simulink model "DEF_2GFL_Eugenie"  (R2022b)
settings: Solver=FixedStepAuto  StartTime=0  StopTime=10  FixedStep=Ts  RelTol=1e-3
undefined symbols (not defined in the file or in its folder): ApparatusDiscreDamping, ApparatusPara, ApparatusPowerFlow, ApparatusType, OtherInputs, PowerFlow, Sbase, Ts, Vbase, Wbase, x_e, Ybase, Zbase
libraries: SimplusGT x10, spsGroundLib x5, spsThreePhaseSeriesRLCBranchLib x4, spsSawtoothGeneratorLib x4, spsabctoAlphaBetaZeroLib x4, spsControlledCurrentSourceLib x3, spsCurrentMeasurementLib x3, spsVoltageMeasurementLib x3, spsThreePhaseParallelRLCBranchLib x2, sps_lib x1
(part 1 of 2)
settings Model: Creator=Maurice  LastModifiedBy=yz34218

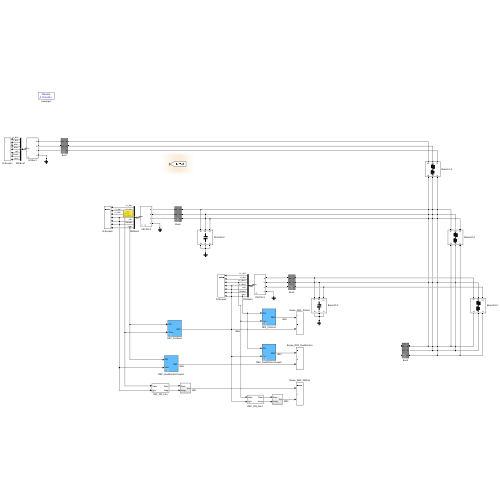
[thumbnail: Simulink's stored preview of the top-level diagram]
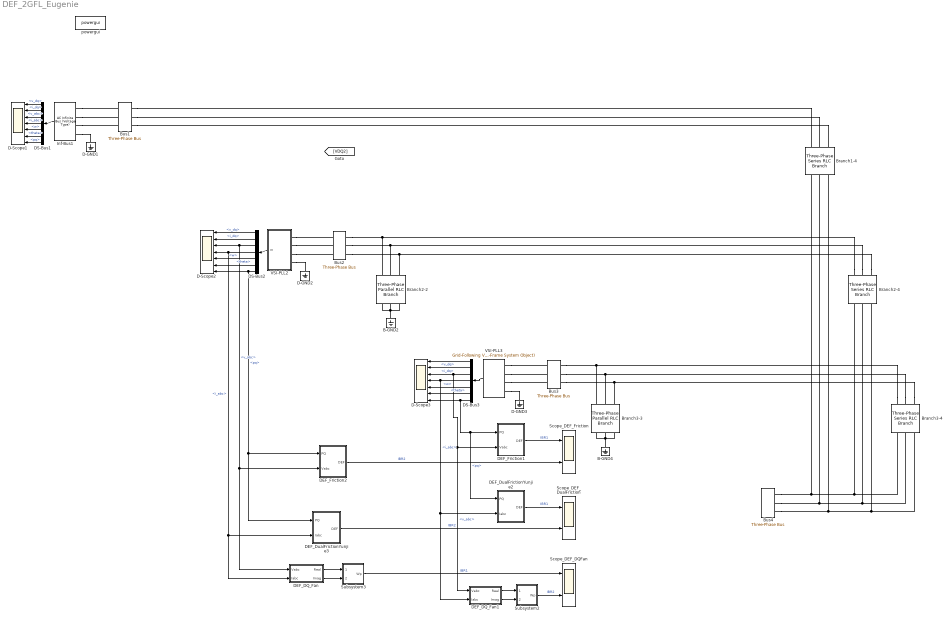
== system DEF_2GFL_Eugenie ==
  B-GND2 : spsGroundLib/Ground  LConnTagsString=a
  B-GND4 : spsGroundLib/Ground  LConnTagsString=a
  Branch1-4 : spsThreePhaseSeriesRLCBranchLib/Three-Phase Series RLC Branch  LConnTagsString=A|B|C  RConnTagsString=A|B|C  BranchType=RL  Resistance=(0.017)*Zbase  Inductance=(0.170)*Zbase/Wbase  Capacitance=1e-6  Measurements=None
  Branch2-2 : spsThreePhaseParallelRLCBranchLib/Three-Phase Parallel RLC Branch  LConnTagsString=A|B|C  RConnTagsString=A|B|C  BranchType=C  Resistance=(Inf)*Zbase  Inductance=(Inf)*Zbase/Wbase  Capacitance=(0.3)*Ybase/Wbase  Measurements=None
  Branch2-4 : spsThreePhaseSeriesRLCBranchLib/Three-Phase Series RLC Branch  LConnTagsString=A|B|C  RConnTagsString=A|B|C  BranchType=RL  Resistance=(0.005)*Zbase  Inductance=(0.05)*Zbase/Wbase  Capacitance=1e-6  Measurements=None
  Branch3-3 : spsThreePhaseParallelRLCBranchLib/Three-Phase Parallel RLC Branch  LConnTagsString=A|B|C  RConnTagsString=A|B|C  BranchType=C  Resistance=(Inf)*Zbase  Inductance=(Inf)*Zbase/Wbase  Capacitance=(0.3)*Ybase/Wbase  Measurements=None
  Branch3-4 : spsThreePhaseSeriesRLCBranchLib/Three-Phase Series RLC Branch  LConnTagsString=A|B|C  RConnTagsString=A|B|C  BranchType=RL  Resistance=(0.005)*Zbase  Inductance=(0.05)*Zbase/Wbase  Capacitance=1e-6  Measurements=None
  Bus{1..4} (4 alike) : SimplusGT/Three-Phase Bus  Vbase=1  Sbase=1
      settings: SourceProductName=Simplus Grid Tool
  D-GND1 : spsGroundLib/Ground  LConnTagsString=a
  D-GND2 : spsGroundLib/Ground  LConnTagsString=a
  D-GND3 : spsGroundLib/Ground  LConnTagsString=a
  D-Scope1 : Scope  NumInputPorts=7
  D-Scope2 : Scope  NumInputPorts=7
  D-Scope3 : Scope  NumInputPorts=7
  DEF_DQ_Fan : Subsystem  mask{PowerFlow_App=ApparatusPowerFlow{2}}
      mask prompts: PowerFlow_App "Power Flow"
  DEF_DQ_Fan1 : Subsystem  mask{PowerFlow_App=ApparatusPowerFlow{3}}
      mask prompts: PowerFlow_App "Power Flow"
  DEF_DualFrictionYunjie2 : Subsystem  mask{PowerFlow_App=ApparatusPowerFlow{3}}
      mask prompts: PowerFlow_App "Power Flow"
  DEF_DualFrictionYunjie3 : Subsystem  mask{PowerFlow_App=ApparatusPowerFlow{3}}
      mask prompts: PowerFlow_App "Power Flow"
  DEF_Friction1 : Subsystem  mask{PowerFlow_App=ApparatusPowerFlow{3}}
      mask prompts: PowerFlow_App "Power Flow"
  DEF_Friction2 : Subsystem  mask{PowerFlow_App=ApparatusPowerFlow{2}}
      mask prompts: PowerFlow_App "Power Flow"
  DS-Bus1 : BusSelector  OutputSignals=v_dq,i_dq,v_abc,i_abc,w,theta,pq
  DS-Bus2 : BusSelector  OutputSignals=v_dq,i_dq,v_abc,i_abc,w,theta,pq
  DS-Bus3 : BusSelector  OutputSignals=v_dq,i_dq,v_abc,i_abc,w,theta,pq
  Inf-Bus1 : SimplusGT/AC Infinite Bus (Voltage Type)  Ts=Ts  Sbase=Sbase  Vbase=Vbase  Wbase=Wbase  vd=PowerFlow{1}(3)  vq=0  theta0=PowerFlow{1}(4)  w=Wbase  R=1e-30
      settings: SourceProductName=Simplus Grid Tool
  Scope_DEF_DQFan : Scope  NumInputPorts=2
  Scope_DEF_DualFriction : Scope  NumInputPorts=2
  Scope_DEF_Friction : Scope  NumInputPorts=2
  Subsystem2 : Subsystem
  Subsystem3 : Subsystem
  VSI-PLL2 : Subsystem  AncestorBlock=|  mask{Ts=Ts, Sbase=Sbase, Vbase=Vbase, Wbase=Wbase, ApparatusType=ApparatusType{2}, ApparatusPara=ApparatusPara{2}, PowerFlow=ApparatusPowerFlow{2}, x0=x_e{2}, OtherInputs=OtherInputs{2}, DiscreMethod=Hybrid Trapezoidal, EnableInsideModification=off, DiscreDampingFlag=on, DiscreDampingValue=ApparatusDiscreDamping{2}, LinearizationTimes=1, DirectFeedthrough=off}
      | SimplusGT/Grid-Following
      | Voltage-Source Inverter
      | (dq-Frame System Object)
      mask prompts: Ts "Ts (s), samping period"; Sbase "Sbase (VA), power base"; Vbase "Vbase (V), voltage base"; Wbase "Wbase (rad/s), frequency base"; ApparatusType "Apparatus type"; ApparatusPara "Apparatus parameters"; PowerFlow "Power flow parameters"; x0 "x0, initial states"; OtherInputs "Other inputs"; DiscreMethod "Discretization method"; EnableInsideModification "Enable inside modification"; DiscreDampingFlag "Enable discretization damping"; DiscreDampingValue "Discretization damping value"; LinearizationTimes "Linearization times"; DirectFeedthrough "Direct feedthrough"
      mask init:
      | SimplusGT.Simulink.DeviceMaskInitialization(EnableInsideModification,DiscreDampingFlag);
      settings: LibrarySourceBlock=|
      | SimplusGT/Grid-Following
      | Voltage-Source Inverter
      | (dq-Frame System Object)
      mask TypeOptions DiscreMethod: Forward Euler | Hybrid Trapezoidal | Virtual Damping
      mask TypeOptions LinearizationTimes: 1 | 2
  VSI-PLL3 : SimplusGT/Grid-Following Voltage-Source Inverter (dq-Frame System Object)  Ts=Ts  Sbase=Sbase  Vbase=Vbase  Wbase=Wbase  ApparatusType=ApparatusType{3}  ApparatusPara=ApparatusPara{3}  PowerFlow=ApparatusPowerFlow{3}  x0=x_e{3}  OtherInputs=OtherInputs{3}  DiscreMethod=Hybrid Trapezoidal  EnableInsideModification=off  DiscreDampingFlag=on  DiscreDampingValue=ApparatusDiscreDamping{3}  LinearizationTimes=1  DirectFeedthrough=off
      settings: SourceProductName=Simplus Grid Tool
  powergui : sps_lib/powergui  Priority=1  SimulationMode=Discrete  SampleTime=Ts  frequency=60  Iterations=50  frequencyindice=0  Pbase=100e6  ErrMax=1e-4  UnitsV=kV  UnitsW=MW  buscounter=0  FunctionMessages=off  echomessages=off  EnableUseOfTLC=off  CurrentSourceSwitches=off  DisableSnubberDevices=off  DisableRonSwitches=off  DisableVfSwitches=off  DisplayEquations=off  AutomaticDiscreteSolvers=off  SolverType=Tustin/Backward Euler (TBE)  Interpol=off  ExternalGateDelay=off  methode=off  Ts=100  x0status=blocks  SPID=on  SwTol=0  HookPort=off  NonlinearTolerance=1e-4  nMaxIteration=100  ContinueOnMaxIteration=off  RestoreLinks=warning  ResistiveCurrentMeasurement=off  Frange=[0:2:500]  Ylog=off  Xlog=on  ShowGrid=off  save=off  variable=ZData  structure=0  ZoomFFT=off  StartTime=0.0  cycles=1  DisplayStyle=1  fundamental=60  FreqAxis=off  MaxFrequency=1000  frequencyindicesteady=1  RmsSteady=1  display=off
  wires:
  Inf-Bus1/1 -> DS-Bus1/1
  DS-Bus1/1 -> D-Scope1/1  "<v_dq>"
  DS-Bus1/2 -> D-Scope1/2  "<i_dq>"
  DS-Bus1/3 -> D-Scope1/3  "<v_abc>"
  DS-Bus1/4 -> D-Scope1/4  "<i_abc>"
  DS-Bus1/5 -> D-Scope1/5  "<w>"
  DS-Bus1/6 -> D-Scope1/6  "<theta>"
  DS-Bus1/7 -> D-Scope1/7  "<pq>"
  DS-Bus2/3 -> DEF_Friction2/2(Vabc), DEF_DQ_Fan/1(Vabc), D-Scope2/3  "<v_abc>"
  DS-Bus2/4 -> DEF_DualFrictionYunjie3/2(Iabc), DEF_DQ_Fan/2(Iabc), D-Scope2/4  "<i_abc>"
  DS-Bus2/5 -> D-Scope2/5  "<w>"
  DS-Bus2/6 -> D-Scope2/6  "<theta>"
  DS-Bus2/7 -> D-Scope2/7, DEF_Friction2/1(PQ), DEF_DualFrictionYunjie3/1(PQ)  "<pq>"
  VSI-PLL3/1 -> DS-Bus3/1
  DS-Bus3/1 -> D-Scope3/1  "<v_dq>"
  DS-Bus3/2 -> D-Scope3/2  "<i_dq>"
  DS-Bus3/3 -> DEF_Friction1/2(Vabc), DEF_DQ_Fan1/1(Vabc), D-Scope3/3  "<v_abc>"
  DS-Bus3/4 -> DEF_DQ_Fan1/2(Iabc), DEF_DualFrictionYunjie2/2(Iabc), D-Scope3/4  "<i_abc>"
  DS-Bus3/5 -> D-Scope3/5  "<w>"
  DS-Bus3/6 -> D-Scope3/6  "<theta>"
  DS-Bus3/7 -> DEF_DualFrictionYunjie2/1(PQ), DEF_Friction1/1(PQ), D-Scope3/7  "<pq>"
  DEF_Friction1/1(DEF) -> Scope_DEF_Friction/1  "IBR1"
  DEF_Friction2/1(DEF) -> Scope_DEF_Friction/2  "IBR2"
  DEF_DualFrictionYunjie2/1(DEF) -> Scope_DEF_DualFriction/1  "IBR1"
  DEF_DualFrictionYunjie3/1(DEF) -> Scope_DEF_DualFriction/2  "IBR2"
  DS-Bus2/2 -> D-Scope2/2  "<i_dq>"
  DS-Bus2/1 -> D-Scope2/1  "<v_dq>"
  DEF_DQ_Fan1/1(Real) -> Subsystem2/1(Real)
  DEF_DQ_Fan1/2(Imag) -> Subsystem2/2(Imag)
  Subsystem2/1(Wp) -> Scope_DEF_DQFan/2  "IBR2"
  DEF_DQ_Fan/2(Imag) -> Subsystem3/2(Imag)
  DEF_DQ_Fan/1(Real) -> Subsystem3/1(Real)
  Subsystem3/1(Wp) -> Scope_DEF_DQFan/1  "IBR1"
  VSI-PLL2/1(m) -> DS-Bus2/1
  connections:
  Inf-Bus1/LConn4 -- D-GND1/LConn1
  VSI-PLL2/LConn4 -- D-GND2/LConn1
  VSI-PLL3/LConn4 -- D-GND3/LConn1
  Branch2-2/RConn1 -- Branch2-2/RConn2 -- Branch2-2/RConn3 -- B-GND2/LConn1
  Branch3-3/RConn1 -- Branch3-3/RConn2 -- Branch3-3/RConn3 -- B-GND4/LConn1
  Branch1-4/RConn1 -- Bus4/RConn1 -- Branch3-4/RConn1 -- Branch2-4/RConn1
  Branch1-4/RConn2 -- Bus4/RConn2 -- Branch3-4/RConn2 -- Branch2-4/RConn2
  Branch1-4/RConn3 -- Bus4/RConn3 -- Branch3-4/RConn3 -- Branch2-4/RConn3
  Bus1/RConn1 -- Branch1-4/LConn1
  Bus1/RConn2 -- Branch1-4/LConn2
  Bus1/RConn3 -- Branch1-4/LConn3
  Branch2-4/LConn1 -- Bus2/RConn1 -- Branch2-2/LConn1
  Branch2-4/LConn2 -- Bus2/RConn2 -- Branch2-2/LConn2
  Branch2-4/LConn3 -- Bus2/RConn3 -- Branch2-2/LConn3
  Branch3-4/LConn1 -- Bus3/RConn1 -- Branch3-3/LConn1
  Branch3-4/LConn2 -- Bus3/RConn2 -- Branch3-3/LConn2
  Branch3-4/LConn3 -- Bus3/RConn3 -- Branch3-3/LConn3
  Inf-Bus1/LConn1 -- Bus1/LConn1
  Inf-Bus1/LConn2 -- Bus1/LConn2
  Inf-Bus1/LConn3 -- Bus1/LConn3
  VSI-PLL2/LConn1 -- Bus2/LConn1
  VSI-PLL2/LConn2 -- Bus2/LConn2
  VSI-PLL2/LConn3 -- Bus2/LConn3
  VSI-PLL3/LConn1 -- Bus3/LConn1
  VSI-PLL3/LConn2 -- Bus3/LConn2
  VSI-PLL3/LConn3 -- Bus3/LConn3

== system DEF_2GFL_Eugenie/DEF_DQ_Fan ==
  Vabc : Inport
  Iabc : Inport  Port=2
  DEF_DualFrictionFan2 : Subsystem
  Mux : Mux  Inputs=2
  Mux1 : Mux  Inputs=2
  dq2DQ : Subsystem
  dq2DQ1 : Subsystem
  Real : Outport
  Imag : Outport  Port=2
  wires:
  Vabc/1 -> dq2DQ/1(abc)
  Iabc/1 -> dq2DQ1/1(abc)
  dq2DQ/1(D) -> Mux/1
  dq2DQ/2(Q) -> Mux/2
  dq2DQ1/1(D) -> Mux1/1
  dq2DQ1/2(Q) -> Mux1/2
  Mux1/1 -> DEF_DualFrictionFan2/2(IDQ)
  Mux/1 -> DEF_DualFrictionFan2/1(VDQ)
  DEF_DualFrictionFan2/1(Real) -> Real/1
  DEF_DualFrictionFan2/2(Imag) -> Imag/1

== system DEF_2GFL_Eugenie/DEF_DQ_Fan1 ==
  Vabc : Inport
  Iabc : Inport  Port=2
  DEF_DualFrictionFan2 : Subsystem
  Mux : Mux  Inputs=2
  Mux1 : Mux  Inputs=2
  dq2DQ : Subsystem
  dq2DQ1 : Subsystem
  Real : Outport
  Imag : Outport  Port=2
  wires:
  DEF_DualFrictionFan2/2(Imag) -> Imag/1
  DEF_DualFrictionFan2/1(Real) -> Real/1
  Mux/1 -> DEF_DualFrictionFan2/1(VDQ)
  Mux1/1 -> DEF_DualFrictionFan2/2(IDQ)
  dq2DQ1/2(Q) -> Mux1/2
  dq2DQ1/1(D) -> Mux1/1
  dq2DQ/2(Q) -> Mux/2
  dq2DQ/1(D) -> Mux/1
  Iabc/1 -> dq2DQ1/1(abc)
  Vabc/1 -> dq2DQ/1(abc)

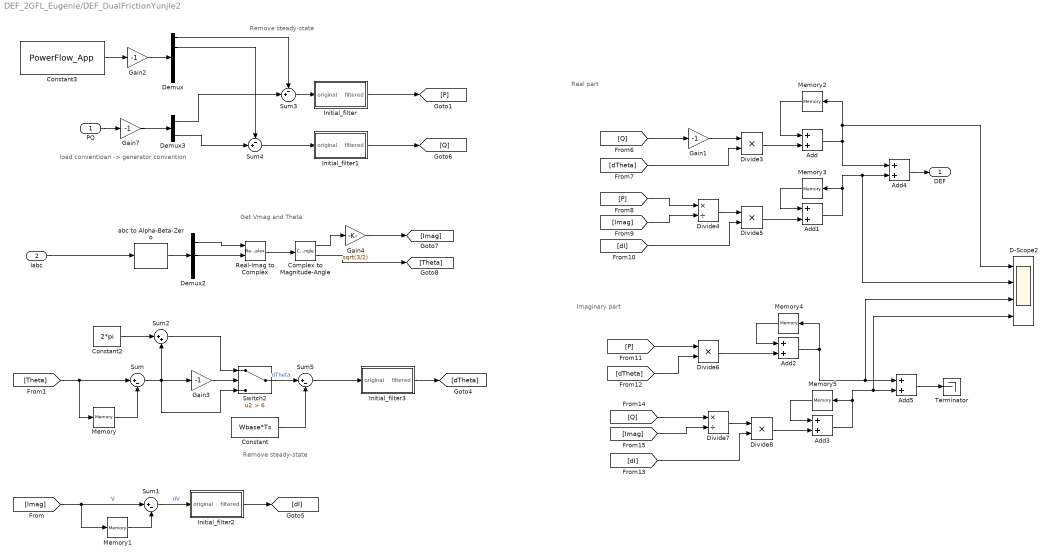
== system DEF_2GFL_Eugenie/DEF_DualFrictionYunjie2 ==
  note: Real part
  note: Imaginary part
  note: load conventioan -> generator convention
  note: Remove steady-state
  note: Remove steady-state
  note: Get Vmag and Theta
  PQ : Inport
  Iabc : Inport  Port=2
  Add{,1..5} (6 alike) : Sum
  Complex to Magnitude-Angle : ComplexToMagnitudeAngle
  Constant : Constant  Value=Wbase*Ts
  Constant2 : Constant  Value=2*pi
  Constant3 : Constant  Value=PowerFlow_App
  D-Scope2 : Scope  NumInputPorts=4
  Demux : Demux  Outputs=5
  Demux2 : Demux  Outputs=3
  Demux3 : Demux  Outputs=2
  Divide{3,5..6,8} (4 alike) : Product  Inputs=**
  Divide4 : Product  Inputs=*/
  Divide7 : Product  Inputs=*/
  Gain{1..3,7} (4 alike) : Gain  Gain=-1
  Gain4 : Gain  Gain=sqrt(3/2)
  Initial_filter : Subsystem
  Initial_filter1 : Subsystem
  Initial_filter2 : Subsystem
  Initial_filter3 : Subsystem
  Memory{,1..5} (6 alike) : Memory
  Real-Imag to Complex : RealImagToComplex
  Sum : Sum  Inputs=|+-
  Sum1 : Sum  Inputs=|+-
  Sum2 : Sum  Inputs=|++
  Sum3 : Sum  Inputs=-+|
  Sum4 : Sum  Inputs=-+|
  Sum5 : Sum  Inputs=|+-
  Switch2 : Switch  Criteria=u2 > Threshold  Threshold=6  SaturateOnIntegerOverflow=off  InputSameDT=off
  Terminator : Terminator
  abc to Alpha-Beta-Zero : spsabctoAlphaBetaZeroLib/abc to Alpha-Beta-Zero
  DEF : Outport
  wires:
  Add4/1 -> DEF/1
  Add5/1 -> Terminator/1
  [Q] -> Divide7/1
  [Imag] -> Divide4/2
  Divide3/1 -> Add/2
  [P] -> Divide4/1
  [Q] -> Gain1/1
  Gain1/1 -> Divide3/1
  [dTheta] -> Divide3/2
  [dI] -> Divide5/2
  [P] -> Divide6/1
  Divide4/1 -> Divide5/1
  [dTheta] -> Divide6/2
  [dI] -> Divide8/2
  Divide7/1 -> Divide8/1
  [Imag] -> Divide7/2
  Memory1/1 -> Sum1/2
  [Imag] -> Memory1/1, Sum1/1  "V"
  Sum1/1 -> Initial_filter2/1(original)  "dV"
  [Theta] -> Sum/1, Memory/1
  Add/1 -> D-Scope2/1, Memory2/1, Add4/1
  Memory2/1 -> Add/1
  Divide5/1 -> Add1/2
  Memory3/1 -> Add1/1
  Memory4/1 -> Add2/1
  Add2/1 -> D-Scope2/3, Add5/1, Memory4/1
  Divide6/1 -> Add2/2
  Memory5/1 -> Add3/1
  Add3/1 -> D-Scope2/4, Add5/2, Memory5/1
  Divide8/1 -> Add3/2
  Iabc/1 -> abc to Alpha-Beta-Zero/1
  abc to Alpha-Beta-Zero/1 -> Demux2/1
  Memory/1 -> Sum/2
  Sum/1 -> Gain3/1, Switch2/3, Sum2/2
  Sum2/1 -> Switch2/1
  Constant2/1 -> Sum2/1
  Gain3/1 -> Switch2/2
  Constant3/1 -> Gain2/1
  Sum3/1 -> Initial_filter/1(original)
  Demux/1 -> Sum3/1
  Sum4/1 -> Initial_filter1/1(original)
  Demux/2 -> Sum4/1
  Demux3/1 -> Sum3/2
  Demux3/2 -> Sum4/2
  PQ/1 -> Gain7/1
  Initial_filter/1(filtered) -> [P]
  Initial_filter1/1(filtered) -> [Q]
  Initial_filter2/1(filtered) -> [dI]
  Initial_filter3/1(filtered) -> [dTheta]
  Complex to Magnitude-Angle/2 -> [Theta]
  Gain4/1 -> [Imag]
  Complex to Magnitude-Angle/1 -> Gain4/1
  Real-Imag to Complex/1 -> Complex to Magnitude-Angle/1
  Demux2/1 -> Real-Imag to Complex/1
  Demux2/2 -> Real-Imag to Complex/2
  Gain2/1 -> Demux/1
  Gain7/1 -> Demux3/1
  Switch2/1 -> Sum5/1  "dTheta"
  Sum5/1 -> Initial_filter3/1(original)
  Constant/1 -> Sum5/2
  Add1/1 -> D-Scope2/2, Add4/2, Memory3/1

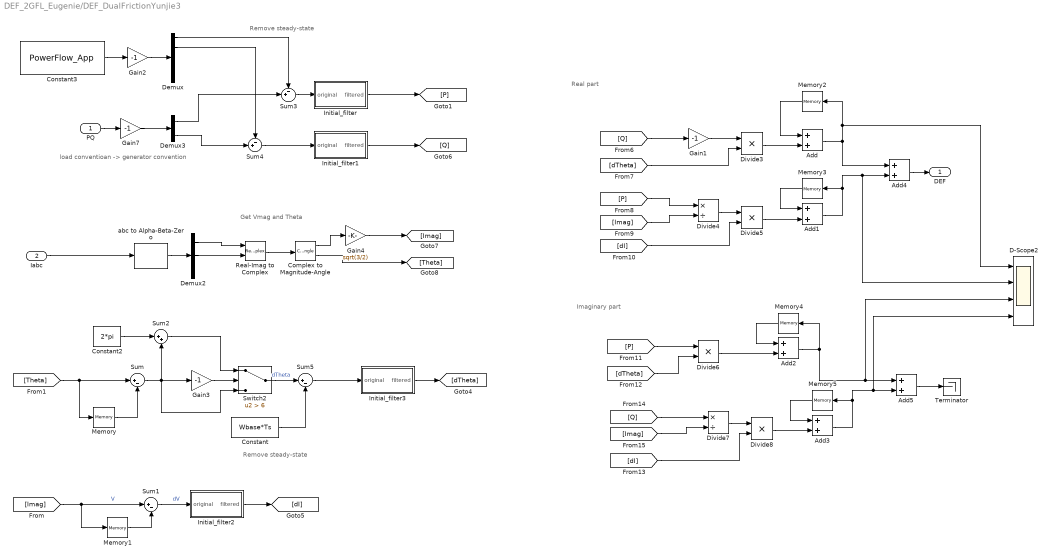
== system DEF_2GFL_Eugenie/DEF_DualFrictionYunjie3 ==
  note: Real part
  note: Imaginary part
  note: load conventioan -> generator convention
  note: Remove steady-state
  note: Remove steady-state
  note: Get Vmag and Theta
  PQ : Inport
  Iabc : Inport  Port=2
  Add{,1..5} (6 alike) : Sum
  Complex to Magnitude-Angle : ComplexToMagnitudeAngle
  Constant : Constant  Value=Wbase*Ts
  Constant2 : Constant  Value=2*pi
  Constant3 : Constant  Value=PowerFlow_App
  D-Scope2 : Scope  NumInputPorts=4
  Demux : Demux  Outputs=5
  Demux2 : Demux  Outputs=3
  Demux3 : Demux  Outputs=2
  Divide{3,5..6,8} (4 alike) : Product  Inputs=**
  Divide4 : Product  Inputs=*/
  Divide7 : Product  Inputs=*/
  Gain{1..3,7} (4 alike) : Gain  Gain=-1
  Gain4 : Gain  Gain=sqrt(3/2)
  Initial_filter : Subsystem
  Initial_filter1 : Subsystem
  Initial_filter2 : Subsystem
  Initial_filter3 : Subsystem
  Memory{,1..5} (6 alike) : Memory
  Real-Imag to Complex : RealImagToComplex
  Sum : Sum  Inputs=|+-
  Sum1 : Sum  Inputs=|+-
  Sum2 : Sum  Inputs=|++
  Sum3 : Sum  Inputs=-+|
  Sum4 : Sum  Inputs=-+|
  Sum5 : Sum  Inputs=|+-
  Switch2 : Switch  Criteria=u2 > Threshold  Threshold=6  SaturateOnIntegerOverflow=off  InputSameDT=off
  Terminator : Terminator
  abc to Alpha-Beta-Zero : spsabctoAlphaBetaZeroLib/abc to Alpha-Beta-Zero
  DEF : Outport
  wires:
  Add4/1 -> DEF/1
  Add5/1 -> Terminator/1
  [Q] -> Divide7/1
  [Imag] -> Divide4/2
  Divide3/1 -> Add/2
  [P] -> Divide4/1
  [Q] -> Gain1/1
  Gain1/1 -> Divide3/1
  [dTheta] -> Divide3/2
  [dI] -> Divide5/2
  [P] -> Divide6/1
  Divide4/1 -> Divide5/1
  [dTheta] -> Divide6/2
  [dI] -> Divide8/2
  Divide7/1 -> Divide8/1
  [Imag] -> Divide7/2
  Memory1/1 -> Sum1/2
  [Imag] -> Memory1/1, Sum1/1  "V"
  Sum1/1 -> Initial_filter2/1(original)  "dV"
  [Theta] -> Sum/1, Memory/1
  Add/1 -> D-Scope2/1, Memory2/1, Add4/1
  Memory2/1 -> Add/1
  Divide5/1 -> Add1/2
  Memory3/1 -> Add1/1
  Memory4/1 -> Add2/1
  Add2/1 -> D-Scope2/3, Add5/1, Memory4/1
  Divide6/1 -> Add2/2
  Memory5/1 -> Add3/1
  Add3/1 -> D-Scope2/4, Add5/2, Memory5/1
  Divide8/1 -> Add3/2
  Iabc/1 -> abc to Alpha-Beta-Zero/1
  abc to Alpha-Beta-Zero/1 -> Demux2/1
  Memory/1 -> Sum/2
  Sum/1 -> Gain3/1, Switch2/3, Sum2/2
  Sum2/1 -> Switch2/1
  Constant2/1 -> Sum2/1
  Gain3/1 -> Switch2/2
  Constant3/1 -> Gain2/1
  Sum3/1 -> Initial_filter/1(original)
  Demux/1 -> Sum3/1
  Sum4/1 -> Initial_filter1/1(original)
  Demux/2 -> Sum4/1
  Demux3/1 -> Sum3/2
  Demux3/2 -> Sum4/2
  PQ/1 -> Gain7/1
  Initial_filter/1(filtered) -> [P]
  Initial_filter1/1(filtered) -> [Q]
  Initial_filter2/1(filtered) -> [dI]
  Initial_filter3/1(filtered) -> [dTheta]
  Complex to Magnitude-Angle/2 -> [Theta]
  Gain4/1 -> [Imag]
  Complex to Magnitude-Angle/1 -> Gain4/1
  Real-Imag to Complex/1 -> Complex to Magnitude-Angle/1
  Demux2/1 -> Real-Imag to Complex/1
  Demux2/2 -> Real-Imag to Complex/2
  Gain2/1 -> Demux/1
  Gain7/1 -> Demux3/1
  Switch2/1 -> Sum5/1  "dTheta"
  Sum5/1 -> Initial_filter3/1(original)
  Constant/1 -> Sum5/2
  Add1/1 -> D-Scope2/2, Add4/2, Memory3/1

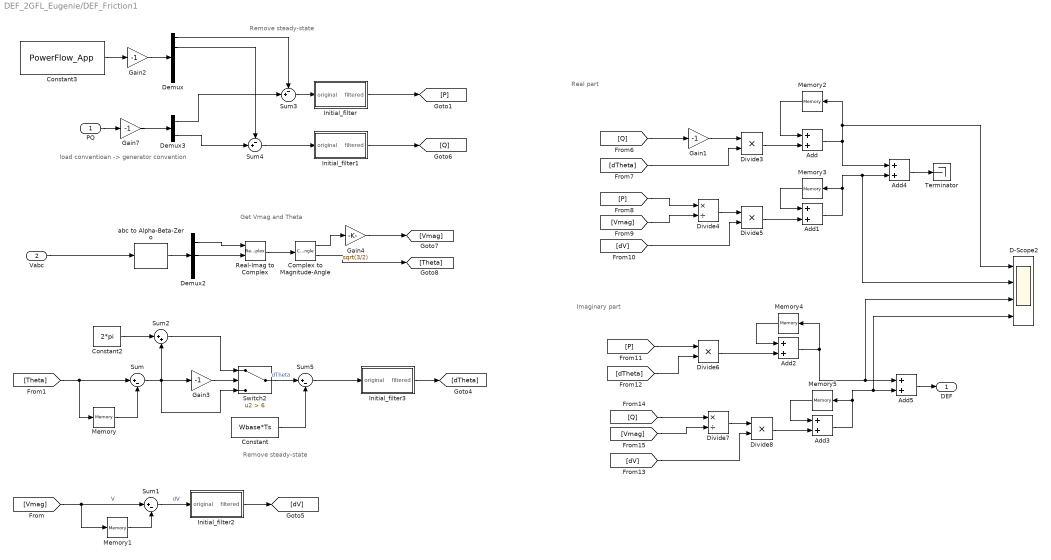
== system DEF_2GFL_Eugenie/DEF_Friction1 ==
  note: Get Vmag and Theta
  note: Remove steady-state
  note: Remove steady-state
  note: load conventioan -> generator convention
  note: Imaginary part
  note: Real part
  PQ : Inport
  Vabc : Inport  Port=2
  Add{,1..5} (6 alike) : Sum
  Complex to Magnitude-Angle : ComplexToMagnitudeAngle
  Constant : Constant  Value=Wbase*Ts
  Constant2 : Constant  Value=2*pi
  Constant3 : Constant  Value=PowerFlow_App
  D-Scope2 : Scope  NumInputPorts=4
  Demux : Demux  Outputs=5
  Demux2 : Demux  Outputs=3
  Demux3 : Demux  Outputs=2
  Divide{3,5..6,8} (4 alike) : Product  Inputs=**
  Divide4 : Product  Inputs=*/
  Divide7 : Product  Inputs=*/
  Gain{1..3,7} (4 alike) : Gain  Gain=-1
  Gain4 : Gain  Gain=sqrt(3/2)
  Initial_filter : Subsystem
  Initial_filter1 : Subsystem
  Initial_filter2 : Subsystem
  Initial_filter3 : Subsystem
  Memory{,1..5} (6 alike) : Memory
  Real-Imag to Complex : RealImagToComplex
  Sum : Sum  Inputs=|+-
  Sum1 : Sum  Inputs=|+-
  Sum2 : Sum  Inputs=|++
  Sum3 : Sum  Inputs=-+|
  Sum4 : Sum  Inputs=-+|
  Sum5 : Sum  Inputs=|+-
  Switch2 : Switch  Criteria=u2 > Threshold  Threshold=6  SaturateOnIntegerOverflow=off  InputSameDT=off
  Terminator : Terminator
  abc to Alpha-Beta-Zero : spsabctoAlphaBetaZeroLib/abc to Alpha-Beta-Zero
  DEF : Outport
  wires:
  Add1/1 -> Memory3/1, Add4/2, D-Scope2/2
  Add4/1 -> Terminator/1
  Add5/1 -> DEF/1
  Constant/1 -> Sum5/2
  Sum5/1 -> Initial_filter3/1(original)
  Switch2/1 -> Sum5/1  "dTheta"
  Gain7/1 -> Demux3/1
  Gain2/1 -> Demux/1
  Demux2/2 -> Real-Imag to Complex/2
  Demux2/1 -> Real-Imag to Complex/1
  Real-Imag to Complex/1 -> Complex to Magnitude-Angle/1
  Complex to Magnitude-Angle/1 -> Gain4/1
  Gain4/1 -> [Vmag]
  Complex to Magnitude-Angle/2 -> [Theta]
  Initial_filter3/1(filtered) -> [dTheta]
  Initial_filter2/1(filtered) -> [dV]
  Initial_filter1/1(filtered) -> [Q]
  Initial_filter/1(filtered) -> [P]
  PQ/1 -> Gain7/1
  Demux3/2 -> Sum4/2
  Demux3/1 -> Sum3/2
  Demux/2 -> Sum4/1
  Sum4/1 -> Initial_filter1/1(original)
  Demux/1 -> Sum3/1
  Sum3/1 -> Initial_filter/1(original)
  Constant3/1 -> Gain2/1
  Gain3/1 -> Switch2/2
  Constant2/1 -> Sum2/1
  Sum2/1 -> Switch2/1
  Sum/1 -> Sum2/2, Switch2/3, Gain3/1
  Memory/1 -> Sum/2
  abc to Alpha-Beta-Zero/1 -> Demux2/1
  Vabc/1 -> abc to Alpha-Beta-Zero/1
  Divide8/1 -> Add3/2
  Add3/1 -> Memory5/1, Add5/2, D-Scope2/4
  Memory5/1 -> Add3/1
  Divide6/1 -> Add2/2
  Add2/1 -> Memory4/1, Add5/1, D-Scope2/3
  Memory4/1 -> Add2/1
  Memory3/1 -> Add1/1
  Divide5/1 -> Add1/2
  Memory2/1 -> Add/1
  Add/1 -> Add4/1, Memory2/1, D-Scope2/1
  [Theta] -> Memory/1, Sum/1
  Sum1/1 -> Initial_filter2/1(original)  "dV"
  [Vmag] -> Sum1/1, Memory1/1  "V"
  Memory1/1 -> Sum1/2
  [Vmag] -> Divide7/2
  Divide7/1 -> Divide8/1
  [dV] -> Divide8/2
  [dTheta] -> Divide6/2
  Divide4/1 -> Divide5/1
  [P] -> Divide6/1
  [dV] -> Divide5/2
  [dTheta] -> Divide3/2
  Gain1/1 -> Divide3/1
  [Q] -> Gain1/1
  [P] -> Divide4/1
  Divide3/1 -> Add/2
  [Vmag] -> Divide4/2
  [Q] -> Divide7/1

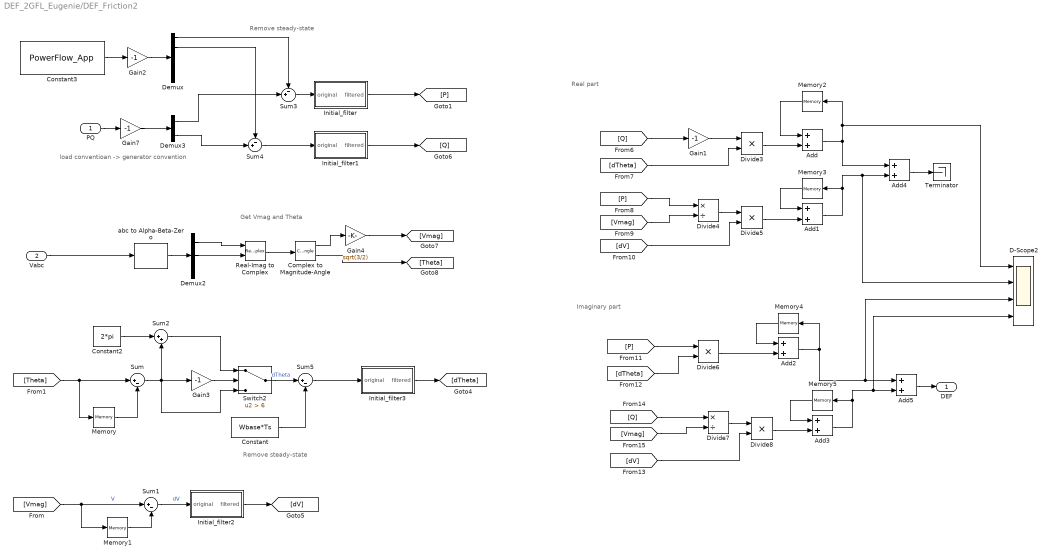
== system DEF_2GFL_Eugenie/DEF_Friction2 ==
  note: Get Vmag and Theta
  note: Remove steady-state
  note: Remove steady-state
  note: load conventioan -> generator convention
  note: Imaginary part
  note: Real part
  PQ : Inport
  Vabc : Inport  Port=2
  Add{,1..5} (6 alike) : Sum
  Complex to Magnitude-Angle : ComplexToMagnitudeAngle
  Constant : Constant  Value=Wbase*Ts
  Constant2 : Constant  Value=2*pi
  Constant3 : Constant  Value=PowerFlow_App
  D-Scope2 : Scope  NumInputPorts=4
  Demux : Demux  Outputs=5
  Demux2 : Demux  Outputs=3
  Demux3 : Demux  Outputs=2
  Divide{3,5..6,8} (4 alike) : Product  Inputs=**
  Divide4 : Product  Inputs=*/
  Divide7 : Product  Inputs=*/
  Gain{1..3,7} (4 alike) : Gain  Gain=-1
  Gain4 : Gain  Gain=sqrt(3/2)
  Initial_filter : Subsystem
  Initial_filter1 : Subsystem
  Initial_filter2 : Subsystem
  Initial_filter3 : Subsystem
  Memory{,1..5} (6 alike) : Memory
  Real-Imag to Complex : RealImagToComplex
  Sum : Sum  Inputs=|+-
  Sum1 : Sum  Inputs=|+-
  Sum2 : Sum  Inputs=|++
  Sum3 : Sum  Inputs=-+|
  Sum4 : Sum  Inputs=-+|
  Sum5 : Sum  Inputs=|+-
  Switch2 : Switch  Criteria=u2 > Threshold  Threshold=6  SaturateOnIntegerOverflow=off  InputSameDT=off
  Terminator : Terminator
  abc to Alpha-Beta-Zero : spsabctoAlphaBetaZeroLib/abc to Alpha-Beta-Zero
  DEF : Outport
  wires:
  Add1/1 -> Memory3/1, Add4/2, D-Scope2/2
  Add4/1 -> Terminator/1
  Add5/1 -> DEF/1
  Constant/1 -> Sum5/2
  Sum5/1 -> Initial_filter3/1(original)
  Switch2/1 -> Sum5/1  "dTheta"
  Gain7/1 -> Demux3/1
  Gain2/1 -> Demux/1
  Demux2/2 -> Real-Imag to Complex/2
  Demux2/1 -> Real-Imag to Complex/1
  Real-Imag to Complex/1 -> Complex to Magnitude-Angle/1
  Complex to Magnitude-Angle/1 -> Gain4/1
  Gain4/1 -> [Vmag]
  Complex to Magnitude-Angle/2 -> [Theta]
  Initial_filter3/1(filtered) -> [dTheta]
  Initial_filter2/1(filtered) -> [dV]
  Initial_filter1/1(filtered) -> [Q]
  Initial_filter/1(filtered) -> [P]
  PQ/1 -> Gain7/1
  Demux3/2 -> Sum4/2
  Demux3/1 -> Sum3/2
  Demux/2 -> Sum4/1
  Sum4/1 -> Initial_filter1/1(original)
  Demux/1 -> Sum3/1
  Sum3/1 -> Initial_filter/1(original)
  Constant3/1 -> Gain2/1
  Gain3/1 -> Switch2/2
  Constant2/1 -> Sum2/1
  Sum2/1 -> Switch2/1
  Sum/1 -> Sum2/2, Switch2/3, Gain3/1
  Memory/1 -> Sum/2
  abc to Alpha-Beta-Zero/1 -> Demux2/1
  Vabc/1 -> abc to Alpha-Beta-Zero/1
  Divide8/1 -> Add3/2
  Add3/1 -> Memory5/1, Add5/2, D-Scope2/4
  Memory5/1 -> Add3/1
  Divide6/1 -> Add2/2
  Add2/1 -> Memory4/1, Add5/1, D-Scope2/3
  Memory4/1 -> Add2/1
  Memory3/1 -> Add1/1
  Divide5/1 -> Add1/2
  Memory2/1 -> Add/1
  Add/1 -> Add4/1, Memory2/1, D-Scope2/1
  [Theta] -> Memory/1, Sum/1
  Sum1/1 -> Initial_filter2/1(original)  "dV"
  [Vmag] -> Sum1/1, Memory1/1  "V"
  Memory1/1 -> Sum1/2
  [Vmag] -> Divide7/2
  Divide7/1 -> Divide8/1
  [dV] -> Divide8/2
  [dTheta] -> Divide6/2
  Divide4/1 -> Divide5/1
  [P] -> Divide6/1
  [dV] -> Divide5/2
  [dTheta] -> Divide3/2
  Gain1/1 -> Divide3/1
  [Q] -> Gain1/1
  [P] -> Divide4/1
  Divide3/1 -> Add/2
  [Vmag] -> Divide4/2
  [Q] -> Divide7/1

== system DEF_2GFL_Eugenie/Subsystem2 ==
  Real : Inport
  Imag : Inport  Port=2
  Add : Sum
  Add1 : Sum
  Constant : Constant  Value=0.1
  Constant1 : Constant
  Math Function : Math  Operator=square
  Product : Product
  Product1 : Product
  Reciprocal Sqrt : Sqrt  Operator=rSqrt
  Wp : Outport
  wires:
  Real/1 -> Product1/1
  Imag/1 -> Add1/1
  Product/1 -> Wp/1
  Math Function/1 -> Add/1
  Reciprocal Sqrt/1 -> Product/2
  Add1/1 -> Product/1
  Constant1/1 -> Add/2
  Constant/1 -> Math Function/1, Product1/2
  Add/1 -> Reciprocal Sqrt/1
  Product1/1 -> Add1/2

== system DEF_2GFL_Eugenie/Subsystem3 ==
  Real : Inport
  Imag : Inport  Port=2
  Add : Sum
  Add1 : Sum
  Constant : Constant  Value=0.1
  Constant1 : Constant
  Math Function : Math  Operator=square
  Product : Product
  Product1 : Product
  Reciprocal Sqrt : Sqrt  Operator=rSqrt
  Wp : Outport
  wires:
  Product1/1 -> Add1/2
  Add/1 -> Reciprocal Sqrt/1
  Constant/1 -> Product1/2, Math Function/1
  Constant1/1 -> Add/2
  Add1/1 -> Product/1
  Reciprocal Sqrt/1 -> Product/2
  Math Function/1 -> Add/1
  Product/1 -> Wp/1
  Imag/1 -> Add1/1
  Real/1 -> Product1/1

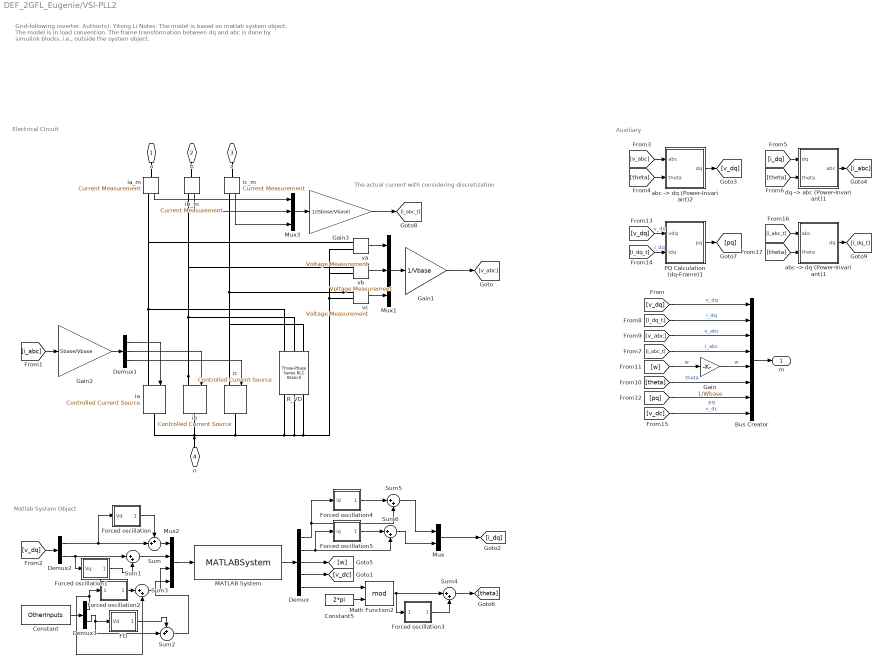
== system DEF_2GFL_Eugenie/VSI-PLL2 ==
  note: The actual current with considering discretization
  note: Grid-following inverter.
      |
      | Author(s): Yitong Li
      |
      | Notes:
      |
      | The model is based on matlab system object.
      |
      | The model is in load convention.
      |
      | The frame transformation between dq and abc is done by simulink blocks, i.e., outside the system object.
  note: Electrical Circuit
  note: Auxiliary
  note: Matlab System Object
  Bus Creator : BusCreator  Inputs=8
  Constant : Constant  Value=OtherInputs
  Constant5 : Constant  Value=2*pi
  Demux : Demux  Outputs=5
  Demux1 : Demux  Outputs=3
  Demux2 : Demux  Outputs=2
  Demux3 : Demux  Outputs=2
  FO : Subsystem
  Forced oscillation : Subsystem
  Forced oscillation1 : Subsystem
  Forced oscillation2 : Subsystem
  Forced oscillation3 : Subsystem
  Forced oscillation4 : Subsystem
  Forced oscillation5 : Subsystem
  Gain : Gain  Gain=1/Wbase
  Gain1 : Gain  Gain=1/Vbase
  Gain2 : Gain  Gain=Sbase/Vbase
  Gain3 : Gain  Gain=1/(Sbase/Vbase)
  MATLAB System : MATLABSystem  System=SimplusGT.Class.GridFollowingVSI  Ts=Ts  Para=ApparatusPara  ApparatusType=ApparatusType  PowerFlow=PowerFlow  x0=x0  DiscreMethod=DiscreMethod  LinearizationTimes=LinearizationTimes  DirectFeedthrough=DirectFeedthrough  VirtualResistor=DiscreDampingFlag  EquiInitial=true  ElecPortIOs=[ 1, 2 ]  SimulateUsing=Code generation
      mask Type: SimplusGT.Class.GridFollowingVSI
      mask Display:
      | disp('GridFollowingVSI');
      | port_label('input',1,'u');
      | port_label('output',1,'y');
  Math Function2 : Math  Operator=mod  SignedPower=on
  Mux : Mux  Inputs=2
  Mux1 : Mux  Inputs=3
  Mux2 : Mux
  Mux3 : Mux  Inputs=3
  PQ Calculation (dq-Frame)1 : Subsystem  AncestorBlock=|
      | SimplusGT/PQ Calculation
      | (dq-Frame)
      settings: LibrarySourceBlock=|
      | SimplusGT/PQ Calculation
      | (dq-Frame)
  R_VD : spsThreePhaseSeriesRLCBranchLib/Three-Phase Series RLC Branch  LConnTagsString=A|B|C  RConnTagsString=A|B|C  BranchType=R  Resistance=DiscreDampingValue*Vbase^2/Sbase  Inductance=1e-3  Capacitance=1e-6  Measurements=None
  Sum : Sum  Inputs=++|
  Sum{1,3..6} (5 alike) : Sum  Inputs=|++
  Sum2 : Sum  Inputs=++|
  "abc -> dq (Power-Invariant)1" : Subsystem  AncestorBlock=|
      | SimplusGT/abc -> dq
      | (Power-Invariant)
      settings: LibrarySourceBlock=|
      | SimplusGT/abc -> dq
      | (Power-Invariant)
  "abc -> dq (Power-Invariant)2" : Subsystem  AncestorBlock=|
      | SimplusGT/abc -> dq
      | (Power-Invariant)
      settings: LibrarySourceBlock=|
      | SimplusGT/abc -> dq
      | (Power-Invariant)
  "dq -> abc (Power-Invariant)1" : Subsystem  AncestorBlock=|
      | SimplusGT/dq -> abc
      | (Power-Invariant)
      settings: LibrarySourceBlock=|
      | SimplusGT/dq -> abc
      | (Power-Invariant)
  ia : spsControlledCurrentSourceLib/Controlled Current Source  Initialize=on  Source_Type=AC  Amplitude=0  Phase=0  Frequency=0  Measurements=None
  ia_m : spsCurrentMeasurementLib/Current Measurement  PhasorSimulation=off  OutputType=Complex  PSBequivalent=0
  ib : spsControlledCurrentSourceLib/Controlled Current Source  Initialize=on  Source_Type=AC  Amplitude=0  Phase=0  Frequency=0  Measurements=None
  ib_m : spsCurrentMeasurementLib/Current Measurement  PhasorSimulation=off  OutputType=Complex  PSBequivalent=0
  ic : spsControlledCurrentSourceLib/Controlled Current Source  Initialize=on  Source_Type=AC  Amplitude=0  Phase=0  Frequency=0  Measurements=None
  ic_m : spsCurrentMeasurementLib/Current Measurement  PhasorSimulation=off  OutputType=Complex  PSBequivalent=0
  va : spsVoltageMeasurementLib/Voltage Measurement  PhasorSimulation=off  OutputType=Complex  PSBequivalent=0
  vb : spsVoltageMeasurementLib/Voltage Measurement  PhasorSimulation=off  OutputType=Complex  PSBequivalent=0
  vc : spsVoltageMeasurementLib/Voltage Measurement  PhasorSimulation=off  OutputType=Complex  PSBequivalent=0
  a : PMIOPort  Side=Left
  b : PMIOPort  Port=2  Side=Left
  c : PMIOPort  Port=3  Side=Left
  n : PMIOPort  Port=4  Side=Left
  m : Outport
  wires:
  "abc -> dq (Power-Invariant)1"/1(dq) -> [i_dq_t]
  [i_abc_t] -> "abc -> dq (Power-Invariant)1"/1(abc)
  [theta] -> "abc -> dq (Power-Invariant)1"/2(theta)
  ia_m/1 -> Mux3/1
  ib_m/1 -> Mux3/2
  Mux3/1 -> Gain3/1
  Gain3/1 -> [i_abc_t]
  ic_m/1 -> Mux3/3
  [v_dc] -> Bus Creator/8  "v_dc"
  Gain1/1 -> [v_abc]
  Gain2/1 -> Demux1/1
  PQ Calculation (dq-Frame)1/1(pq) -> [pq]
  [i_dq_t] -> PQ Calculation (dq-Frame)1/2(idq)  "i_dq"
  [v_dq] -> PQ Calculation (dq-Frame)1/1(vdq)  "v_dq"
  [pq] -> Bus Creator/7  "pq"
  [i_abc] -> Gain2/1
  Gain/1 -> Bus Creator/5  "w"
  [w] -> Gain/1  "w"
  Constant/1 -> Demux3/1
  Bus Creator/1 -> m/1
  Demux/4 -> [v_dc]
  Math Function2/1 -> Sum4/1, Forced oscillation3/1(theta)
  Constant5/1 -> Math Function2/2
  Demux/5 -> Math Function2/1
  Demux1/3 -> ic/1
  vc/1 -> Mux1/3
  MATLAB System/1 -> Demux/1
  Mux2/1 -> MATLAB System/1
  "dq -> abc (Power-Invariant)1"/1(abc) -> [i_abc]
  [theta] -> "dq -> abc (Power-Invariant)1"/2(theta)
  [i_dq] -> "dq -> abc (Power-Invariant)1"/1(dq)
  "abc -> dq (Power-Invariant)2"/1(dq) -> [v_dq]
  [theta] -> "abc -> dq (Power-Invariant)2"/2(theta)
  [v_abc] -> "abc -> dq (Power-Invariant)2"/1(abc)
  [theta] -> Bus Creator/6  "theta"
  [i_abc_t] -> Bus Creator/4  "i_abc"
  [v_abc] -> Bus Creator/3  "v_abc"
  [i_dq_t] -> Bus Creator/2  "i_dq"
  [v_dq] -> Bus Creator/1  "v_dq"
  Demux2/1 -> Forced oscillation/1(Vd), Sum/2
  [v_dq] -> Demux2/1
  Mux1/1 -> Gain1/1
  vb/1 -> Mux1/2
  va/1 -> Mux1/1
  Demux1/2 -> ib/1
  Demux1/1 -> ia/1
  Demux/3 -> [w]
  Mux/1 -> [i_dq]
  Demux/2 -> Sum6/2, Forced oscillation5/1(iq)
  Sum/1 -> Mux2/1
  Forced oscillation/1(Out1) -> Sum/1
  Forced oscillation1/1(Out1) -> Sum1/2
  Demux2/2 -> Sum1/1, Forced oscillation1/1(Vq)
  Sum1/1 -> Mux2/2
  Demux3/1 -> Sum3/2, Forced oscillation2/1(angr)
  Demux3/2 -> Sum2/2, FO/1(Vd)
  FO/1(Out1) -> Sum2/1
  Sum2/1 -> Mux2/4
  Forced oscillation2/1(Out1) -> Sum3/1
  Sum3/1 -> Mux2/3
  Sum4/1 -> [theta]
  Forced oscillation3/1(Out1) -> Sum4/2
  Forced oscillation4/1(Out1) -> Sum5/1
  Demux/1 -> Sum5/2, Forced oscillation4/1(id)
  Sum5/1 -> Mux/1
  Forced oscillation5/1(Out1) -> Sum6/1
  Sum6/1 -> Mux/2
  connections:
  ia_m/LConn1 -- a/RConn1
  ib_m/LConn1 -- b/RConn1
  ic_m/LConn1 -- c/RConn1
  vc/LConn1 -- ic_m/RConn1 -- ic/LConn1 -- R_VD/LConn3
  ib/LConn1 -- vb/LConn1 -- ib_m/RConn1 -- R_VD/LConn2
  ia/LConn1 -- ia_m/RConn1 -- va/LConn1 -- R_VD/LConn1
  n/RConn1 -- ib/RConn1 -- ia/RConn1 -- ic/RConn1 -- R_VD/RConn1 -- R_VD/RConn2 -- R_VD/RConn3 -- vc/LConn2 -- va/LConn2 -- vb/LConn2

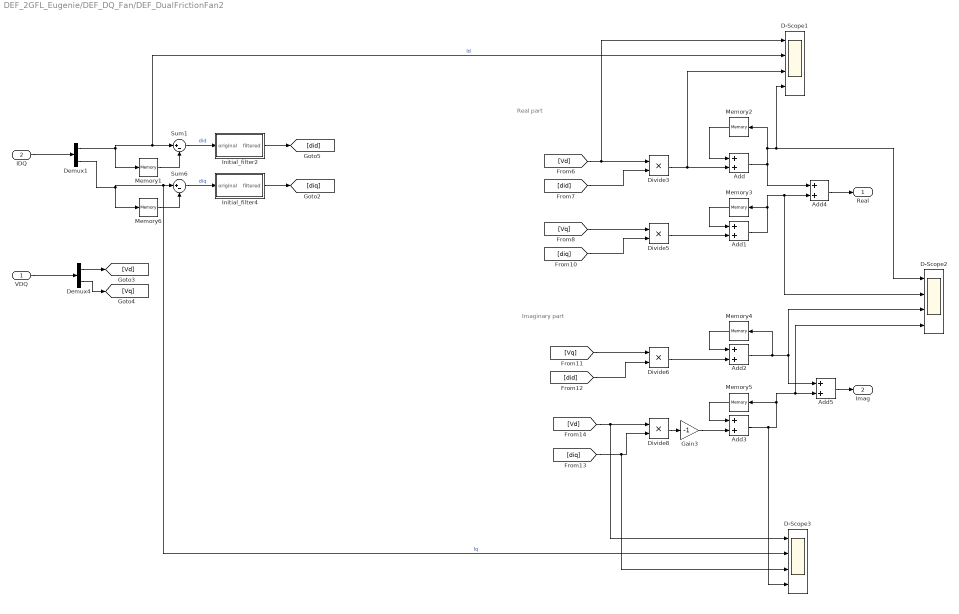
== system DEF_2GFL_Eugenie/DEF_DQ_Fan/DEF_DualFrictionFan2 ==
  note: Real part
  note: Imaginary part
  VDQ : Inport
  IDQ : Inport  Port=2
  Add{,1..5} (6 alike) : Sum
  D-Scope1 : Scope  NumInputPorts=4
  D-Scope2 : Scope  NumInputPorts=4
  D-Scope3 : Scope  NumInputPorts=4
  Demux1 : Demux  Outputs=2
  Demux4 : Demux  Outputs=2
  Divide{3,5..6,8} (4 alike) : Product  Inputs=**
  Gain3 : Gain  Gain=-1
  Initial_filter2 : Subsystem
  Initial_filter4 : Subsystem
  Memory{1..6} (6 alike) : Memory
  Sum1 : Sum  Inputs=|+-
  Sum6 : Sum  Inputs=|+-
  Real : Outport
  Imag : Outport  Port=2
  wires:
  Add5/1 -> Imag/1
  Add4/1 -> Real/1
  Gain3/1 -> Add3/2
  Demux4/2 -> [Vq]
  Demux4/1 -> [Vd]
  Initial_filter4/1(filtered) -> [diq]
  Sum6/1 -> Initial_filter4/1(original)  "diq"
  Demux1/2 -> Sum6/1, D-Scope3/2, Memory6/1  "Iq"
  Memory6/1 -> Sum6/2
  Divide3/1 -> Add/2, D-Scope1/3
  [Vd] -> Divide3/1, D-Scope1/1
  [did] -> Divide3/2
  [diq] -> Divide5/2
  [Vq] -> Divide6/1
  [Vq] -> Divide5/1
  [did] -> Divide6/2
  [diq] -> Divide8/2, D-Scope3/3
  [Vd] -> Divide8/1, D-Scope3/1
  Memory1/1 -> Sum1/2
  Demux1/1 -> Memory1/1, Sum1/1, D-Scope1/2  "Id"
  Sum1/1 -> Initial_filter2/1(original)  "did"
  Add/1 -> D-Scope2/1, D-Scope1/4, Memory2/1, Add4/1
  Memory2/1 -> Add/1
  Divide5/1 -> Add1/2
  Memory3/1 -> Add1/1
  Memory4/1 -> Add2/1
  Add2/1 -> D-Scope2/3, Add5/1, Memory4/1
  Divide6/1 -> Add2/2
  Memory5/1 -> Add3/1
  Add3/1 -> D-Scope2/4, Add5/2, Memory5/1, D-Scope3/4
  Divide8/1 -> Gain3/1
  IDQ/1 -> Demux1/1
  VDQ/1 -> Demux4/1
  Initial_filter2/1(filtered) -> [did]
  Add1/1 -> D-Scope2/2, Add4/2, Memory3/1

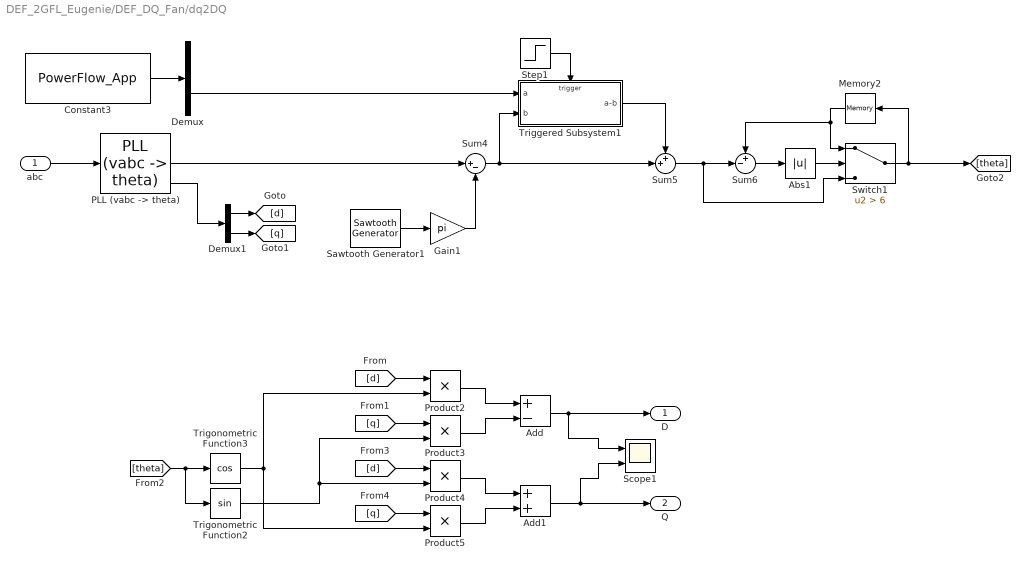
== system DEF_2GFL_Eugenie/DEF_DQ_Fan/dq2DQ ==
  abc : Inport
  Abs1 : Abs  SaturateOnIntegerOverflow=off
  Add : Sum  Inputs=+-
  Add1 : Sum
  Constant3 : Constant  Value=PowerFlow_App
  Demux : Demux  Outputs=5
  Demux1 : Demux  Outputs=2
  Gain1 : Gain  Gain=pi
  Memory2 : Memory
  "PLL (vabc -> theta)" : SimplusGT/PLL (vabc -> theta)  Ts=Ts  Wbase=Wbase  w_pll=5  w_tau=300  theta0=0.1277
      settings: SourceProductName=Simplus Grid Tool
  Product{2..5} (4 alike) : Product
  Sawtooth Generator1 : spsSawtoothGeneratorLib/Sawtooth Generator  Freq=50  Phase=180  Ts=0
  Scope1 : Scope  NumInputPorts=2
  Step1 : Step  SampleTime=0
  Sum4 : Sum  Inputs=|+-
  Sum5 : Sum  Inputs=++|
  Sum6 : Sum  Inputs=+-|
  Switch1 : Switch  Criteria=u2 > Threshold  Threshold=6  SaturateOnIntegerOverflow=off  InputSameDT=off
  Triggered Subsystem1 : Subsystem  TreatAsAtomicUnit=on
  Trigonometric Function2 : Trigonometry
  Trigonometric Function3 : Trigonometry  Operator=cos
  D : Outport
  Q : Outport  Port=2
  wires:
  Demux1/1 -> [d]
  Demux/4 -> Triggered Subsystem1/1(a)
  Sum4/1 -> Triggered Subsystem1/2(b), Sum5/2
  Product3/1 -> Add/2
  Add/1 -> D/1, Scope1/1
  Trigonometric Function2/1 -> Product4/2, Product3/2
  Step1/1 -> Triggered Subsystem1/Trigger
  [theta] -> Trigonometric Function2/1, Trigonometric Function3/1
  Add1/1 -> Q/1, Scope1/2
  Sum5/1 -> Switch1/3, Sum6/2
  Triggered Subsystem1/1(a-b) -> Sum5/1
  Sawtooth Generator1/1 -> Gain1/1
  [q] -> Product5/1
  abc/1 -> "PLL (vabc -> theta)"/1
  Memory2/1 -> Switch1/1, Sum6/1
  Switch1/1 -> Memory2/1, [theta]
  Trigonometric Function3/1 -> Product2/2, Product5/2
  Sum6/1 -> Abs1/1
  Product5/1 -> Add1/2
  Product2/1 -> Add/1
  "PLL (vabc -> theta)"/2 -> Sum4/1
  Product4/1 -> Add1/1
  "PLL (vabc -> theta)"/3 -> Demux1/1
  Abs1/1 -> Switch1/2
  Demux1/2 -> [q]
  [d] -> Product4/1
  [q] -> Product3/1
  [d] -> Product2/1
  Constant3/1 -> Demux/1
  Gain1/1 -> Sum4/2

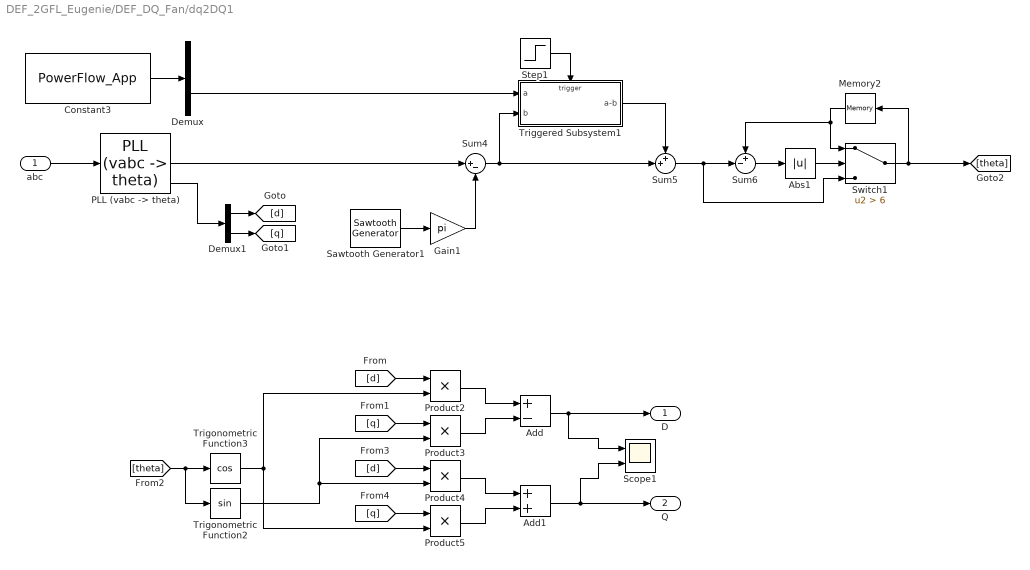
== system DEF_2GFL_Eugenie/DEF_DQ_Fan/dq2DQ1 ==
  abc : Inport
  Abs1 : Abs  SaturateOnIntegerOverflow=off
  Add : Sum  Inputs=+-
  Add1 : Sum
  Constant3 : Constant  Value=PowerFlow_App
  Demux : Demux  Outputs=5
  Demux1 : Demux  Outputs=2
  Gain1 : Gain  Gain=pi
  Memory2 : Memory
  "PLL (vabc -> theta)" : SimplusGT/PLL (vabc -> theta)  Ts=Ts  Wbase=Wbase  w_pll=5  w_tau=300  theta0=0.1277
      settings: SourceProductName=Simplus Grid Tool
  Product{2..5} (4 alike) : Product
  Sawtooth Generator1 : spsSawtoothGeneratorLib/Sawtooth Generator  Freq=50  Phase=180  Ts=0
  Scope1 : Scope  NumInputPorts=2
  Step1 : Step  SampleTime=0
  Sum4 : Sum  Inputs=|+-
  Sum5 : Sum  Inputs=++|
  Sum6 : Sum  Inputs=+-|
  Switch1 : Switch  Criteria=u2 > Threshold  Threshold=6  SaturateOnIntegerOverflow=off  InputSameDT=off
  Triggered Subsystem1 : Subsystem  TreatAsAtomicUnit=on
  Trigonometric Function2 : Trigonometry
  Trigonometric Function3 : Trigonometry  Operator=cos
  D : Outport
  Q : Outport  Port=2
  wires:
  Gain1/1 -> Sum4/2
  Constant3/1 -> Demux/1
  [d] -> Product2/1
  [q] -> Product3/1
  [d] -> Product4/1
  Demux1/2 -> [q]
  Abs1/1 -> Switch1/2
  "PLL (vabc -> theta)"/3 -> Demux1/1
  Product4/1 -> Add1/1
  "PLL (vabc -> theta)"/2 -> Sum4/1
  Product2/1 -> Add/1
  Product5/1 -> Add1/2
  Sum6/1 -> Abs1/1
  Trigonometric Function3/1 -> Product5/2, Product2/2
  Switch1/1 -> [theta], Memory2/1
  Memory2/1 -> Sum6/1, Switch1/1
  abc/1 -> "PLL (vabc -> theta)"/1
  [q] -> Product5/1
  Sawtooth Generator1/1 -> Gain1/1
  Triggered Subsystem1/1(a-b) -> Sum5/1
  Sum5/1 -> Sum6/2, Switch1/3
  Add1/1 -> Scope1/2, Q/1
  [theta] -> Trigonometric Function3/1, Trigonometric Function2/1
  Step1/1 -> Triggered Subsystem1/Trigger
  Trigonometric Function2/1 -> Product3/2, Product4/2
  Add/1 -> Scope1/1, D/1
  Product3/1 -> Add/2
  Sum4/1 -> Sum5/2, Triggered Subsystem1/2(b)
  Demux/4 -> Triggered Subsystem1/1(a)
  Demux1/1 -> [d]

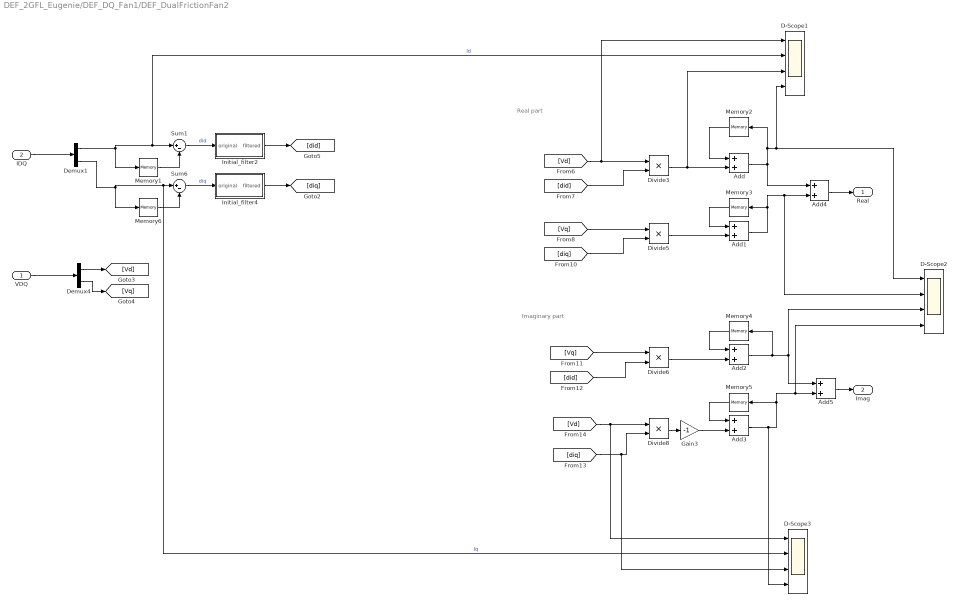
== system DEF_2GFL_Eugenie/DEF_DQ_Fan1/DEF_DualFrictionFan2 ==
  note: Imaginary part
  note: Real part
  VDQ : Inport
  IDQ : Inport  Port=2
  Add{,1..5} (6 alike) : Sum
  D-Scope1 : Scope  NumInputPorts=4
  D-Scope2 : Scope  NumInputPorts=4
  D-Scope3 : Scope  NumInputPorts=4
  Demux1 : Demux  Outputs=2
  Demux4 : Demux  Outputs=2
  Divide{3,5..6,8} (4 alike) : Product  Inputs=**
  Gain3 : Gain  Gain=-1
  Initial_filter2 : Subsystem
  Initial_filter4 : Subsystem
  Memory{1..6} (6 alike) : Memory
  Sum1 : Sum  Inputs=|+-
  Sum6 : Sum  Inputs=|+-
  Real : Outport
  Imag : Outport  Port=2
  wires:
  Add1/1 -> Memory3/1, Add4/2, D-Scope2/2
  Initial_filter2/1(filtered) -> [did]
  VDQ/1 -> Demux4/1
  IDQ/1 -> Demux1/1
  Divide8/1 -> Gain3/1
  Add3/1 -> D-Scope3/4, Memory5/1, Add5/2, D-Scope2/4
  Memory5/1 -> Add3/1
  Divide6/1 -> Add2/2
  Add2/1 -> Memory4/1, Add5/1, D-Scope2/3
  Memory4/1 -> Add2/1
  Memory3/1 -> Add1/1
  Divide5/1 -> Add1/2
  Memory2/1 -> Add/1
  Add/1 -> Add4/1, Memory2/1, D-Scope1/4, D-Scope2/1
  Sum1/1 -> Initial_filter2/1(original)  "did"
  Demux1/1 -> D-Scope1/2, Sum1/1, Memory1/1  "Id"
  Memory1/1 -> Sum1/2
  [Vd] -> D-Scope3/1, Divide8/1
  [diq] -> D-Scope3/3, Divide8/2
  [did] -> Divide6/2
  [Vq] -> Divide5/1
  [Vq] -> Divide6/1
  [diq] -> Divide5/2
  [did] -> Divide3/2
  [Vd] -> D-Scope1/1, Divide3/1
  Divide3/1 -> D-Scope1/3, Add/2
  Memory6/1 -> Sum6/2
  Demux1/2 -> Memory6/1, D-Scope3/2, Sum6/1  "Iq"
  Sum6/1 -> Initial_filter4/1(original)  "diq"
  Initial_filter4/1(filtered) -> [diq]
  Demux4/1 -> [Vd]
  Demux4/2 -> [Vq]
  Gain3/1 -> Add3/2
  Add4/1 -> Real/1
  Add5/1 -> Imag/1

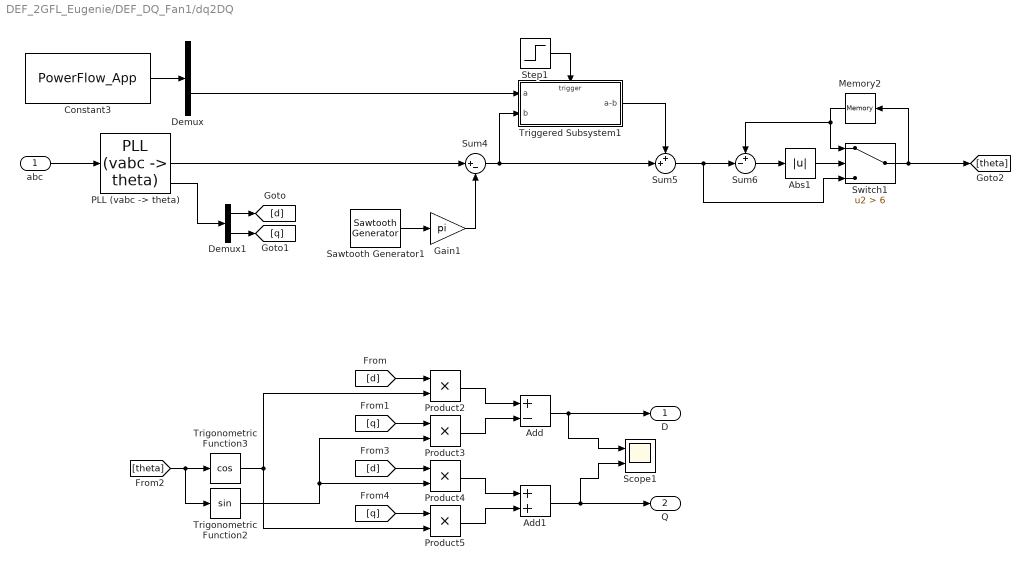
== system DEF_2GFL_Eugenie/DEF_DQ_Fan1/dq2DQ ==
  abc : Inport
  Abs1 : Abs  SaturateOnIntegerOverflow=off
  Add : Sum  Inputs=+-
  Add1 : Sum
  Constant3 : Constant  Value=PowerFlow_App
  Demux : Demux  Outputs=5
  Demux1 : Demux  Outputs=2
  Gain1 : Gain  Gain=pi
  Memory2 : Memory
  "PLL (vabc -> theta)" : SimplusGT/PLL (vabc -> theta)  Ts=Ts  Wbase=Wbase  w_pll=5  w_tau=300  theta0=0.1277
      settings: SourceProductName=Simplus Grid Tool
  Product{2..5} (4 alike) : Product
  Sawtooth Generator1 : spsSawtoothGeneratorLib/Sawtooth Generator  Freq=50  Phase=180  Ts=0
  Scope1 : Scope  NumInputPorts=2
  Step1 : Step  SampleTime=0
  Sum4 : Sum  Inputs=|+-
  Sum5 : Sum  Inputs=++|
  Sum6 : Sum  Inputs=+-|
  Switch1 : Switch  Criteria=u2 > Threshold  Threshold=6  SaturateOnIntegerOverflow=off  InputSameDT=off
  Triggered Subsystem1 : Subsystem  TreatAsAtomicUnit=on
  Trigonometric Function2 : Trigonometry
  Trigonometric Function3 : Trigonometry  Operator=cos
  D : Outport
  Q : Outport  Port=2
  wires:
  Gain1/1 -> Sum4/2
  Constant3/1 -> Demux/1
  [d] -> Product2/1
  [q] -> Product3/1
  [d] -> Product4/1
  Demux1/2 -> [q]
  Abs1/1 -> Switch1/2
  "PLL (vabc -> theta)"/3 -> Demux1/1
  Product4/1 -> Add1/1
  "PLL (vabc -> theta)"/2 -> Sum4/1
  Product2/1 -> Add/1
  Product5/1 -> Add1/2
  Sum6/1 -> Abs1/1
  Trigonometric Function3/1 -> Product5/2, Product2/2
  Switch1/1 -> [theta], Memory2/1
  Memory2/1 -> Sum6/1, Switch1/1
  abc/1 -> "PLL (vabc -> theta)"/1
  [q] -> Product5/1
  Sawtooth Generator1/1 -> Gain1/1
  Triggered Subsystem1/1(a-b) -> Sum5/1
  Sum5/1 -> Sum6/2, Switch1/3
  Add1/1 -> Scope1/2, Q/1
  [theta] -> Trigonometric Function3/1, Trigonometric Function2/1
  Step1/1 -> Triggered Subsystem1/Trigger
  Trigonometric Function2/1 -> Product3/2, Product4/2
  Add/1 -> Scope1/1, D/1
  Product3/1 -> Add/2
  Sum4/1 -> Sum5/2, Triggered Subsystem1/2(b)
  Demux/4 -> Triggered Subsystem1/1(a)
  Demux1/1 -> [d]

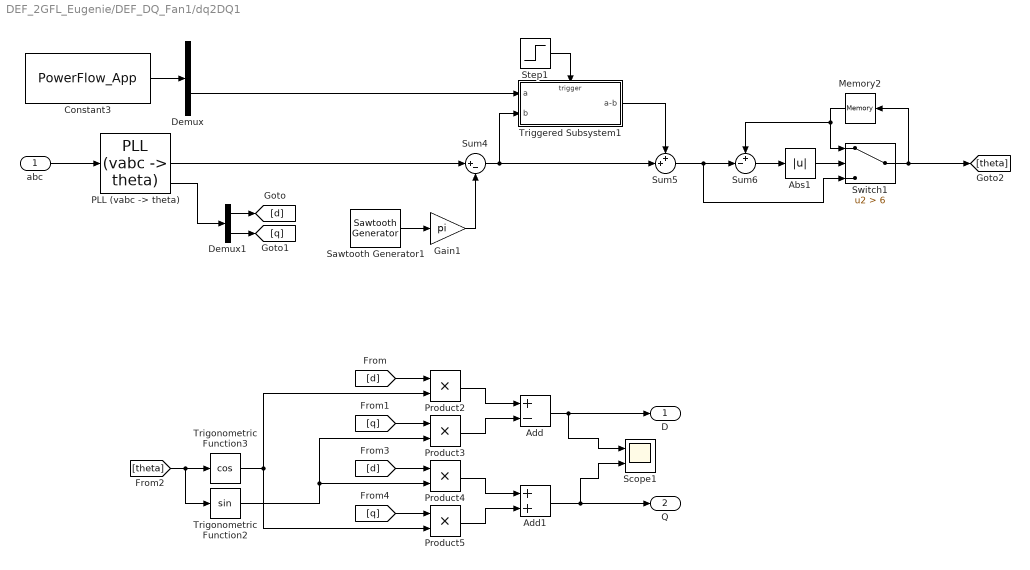
== system DEF_2GFL_Eugenie/DEF_DQ_Fan1/dq2DQ1 ==
  abc : Inport
  Abs1 : Abs  SaturateOnIntegerOverflow=off
  Add : Sum  Inputs=+-
  Add1 : Sum
  Constant3 : Constant  Value=PowerFlow_App
  Demux : Demux  Outputs=5
  Demux1 : Demux  Outputs=2
  Gain1 : Gain  Gain=pi
  Memory2 : Memory
  "PLL (vabc -> theta)" : SimplusGT/PLL (vabc -> theta)  Ts=Ts  Wbase=Wbase  w_pll=5  w_tau=300  theta0=0.1277
      settings: SourceProductName=Simplus Grid Tool
  Product{2..5} (4 alike) : Product
  Sawtooth Generator1 : spsSawtoothGeneratorLib/Sawtooth Generator  Freq=50  Phase=180  Ts=0
  Scope1 : Scope  NumInputPorts=2
  Step1 : Step  SampleTime=0
  Sum4 : Sum  Inputs=|+-
  Sum5 : Sum  Inputs=++|
  Sum6 : Sum  Inputs=+-|
  Switch1 : Switch  Criteria=u2 > Threshold  Threshold=6  SaturateOnIntegerOverflow=off  InputSameDT=off
  Triggered Subsystem1 : Subsystem  TreatAsAtomicUnit=on
  Trigonometric Function2 : Trigonometry
  Trigonometric Function3 : Trigonometry  Operator=cos
  D : Outport
  Q : Outport  Port=2
  wires:
  Demux1/1 -> [d]
  Demux/4 -> Triggered Subsystem1/1(a)
  Sum4/1 -> Triggered Subsystem1/2(b), Sum5/2
  Product3/1 -> Add/2
  Add/1 -> D/1, Scope1/1
  Trigonometric Function2/1 -> Product4/2, Product3/2
  Step1/1 -> Triggered Subsystem1/Trigger
  [theta] -> Trigonometric Function2/1, Trigonometric Function3/1
  Add1/1 -> Q/1, Scope1/2
  Sum5/1 -> Switch1/3, Sum6/2
  Triggered Subsystem1/1(a-b) -> Sum5/1
  Sawtooth Generator1/1 -> Gain1/1
  [q] -> Product5/1
  abc/1 -> "PLL (vabc -> theta)"/1
  Memory2/1 -> Switch1/1, Sum6/1
  Switch1/1 -> Memory2/1, [theta]
  Trigonometric Function3/1 -> Product2/2, Product5/2
  Sum6/1 -> Abs1/1
  Product5/1 -> Add1/2
  Product2/1 -> Add/1
  "PLL (vabc -> theta)"/2 -> Sum4/1
  Product4/1 -> Add1/1
  "PLL (vabc -> theta)"/3 -> Demux1/1
  Abs1/1 -> Switch1/2
  Demux1/2 -> [q]
  [d] -> Product4/1
  [q] -> Product3/1
  [d] -> Product2/1
  Constant3/1 -> Demux/1
  Gain1/1 -> Sum4/2

== system DEF_2GFL_Eugenie/DEF_DualFrictionYunjie2/Initial_filter ==
  original : Inport
  Clock1 : Clock
  Gain7 : Gain
  Gain8 : Gain  Gain=0
  Switch3 : Switch  Criteria=u2 > Threshold  Threshold=1.5  SaturateOnIntegerOverflow=off  InputSameDT=off
  filtered : Outport
  wires:
  Switch3/1 -> filtered/1  "dTheta"
  original/1 -> Gain8/1, Gain7/1
  Gain7/1 -> Switch3/1
  Gain8/1 -> Switch3/3
  Clock1/1 -> Switch3/2

== system DEF_2GFL_Eugenie/DEF_DualFrictionYunjie2/Initial_filter1 ==
  original : Inport
  Clock1 : Clock
  Gain7 : Gain
  Gain8 : Gain  Gain=0
  Switch3 : Switch  Criteria=u2 > Threshold  Threshold=1.5  SaturateOnIntegerOverflow=off  InputSameDT=off
  filtered : Outport
  wires:
  Switch3/1 -> filtered/1  "dTheta"
  original/1 -> Gain8/1, Gain7/1
  Gain7/1 -> Switch3/1
  Gain8/1 -> Switch3/3
  Clock1/1 -> Switch3/2

== system DEF_2GFL_Eugenie/DEF_DualFrictionYunjie2/Initial_filter2 ==
  original : Inport
  Clock1 : Clock
  Gain7 : Gain
  Gain8 : Gain  Gain=0
  Switch3 : Switch  Criteria=u2 > Threshold  Threshold=1.5  SaturateOnIntegerOverflow=off  InputSameDT=off
  filtered : Outport
  wires:
  Switch3/1 -> filtered/1  "dTheta"
  original/1 -> Gain8/1, Gain7/1
  Gain7/1 -> Switch3/1
  Gain8/1 -> Switch3/3
  Clock1/1 -> Switch3/2

== system DEF_2GFL_Eugenie/DEF_DualFrictionYunjie2/Initial_filter3 ==
  original : Inport
  Clock1 : Clock
  Gain7 : Gain
  Gain8 : Gain  Gain=0
  Switch3 : Switch  Criteria=u2 > Threshold  Threshold=1.5  SaturateOnIntegerOverflow=off  InputSameDT=off
  filtered : Outport
  wires:
  Switch3/1 -> filtered/1  "dTheta"
  original/1 -> Gain8/1, Gain7/1
  Gain7/1 -> Switch3/1
  Gain8/1 -> Switch3/3
  Clock1/1 -> Switch3/2

== system DEF_2GFL_Eugenie/DEF_DualFrictionYunjie3/Initial_filter ==
  original : Inport
  Clock1 : Clock
  Gain7 : Gain
  Gain8 : Gain  Gain=0
  Switch3 : Switch  Criteria=u2 > Threshold  Threshold=1.5  SaturateOnIntegerOverflow=off  InputSameDT=off
  filtered : Outport
  wires:
  Switch3/1 -> filtered/1  "dTheta"
  original/1 -> Gain8/1, Gain7/1
  Gain7/1 -> Switch3/1
  Gain8/1 -> Switch3/3
  Clock1/1 -> Switch3/2

== system DEF_2GFL_Eugenie/DEF_DualFrictionYunjie3/Initial_filter1 ==
  original : Inport
  Clock1 : Clock
  Gain7 : Gain
  Gain8 : Gain  Gain=0
  Switch3 : Switch  Criteria=u2 > Threshold  Threshold=1.5  SaturateOnIntegerOverflow=off  InputSameDT=off
  filtered : Outport
  wires:
  Switch3/1 -> filtered/1  "dTheta"
  original/1 -> Gain8/1, Gain7/1
  Gain7/1 -> Switch3/1
  Gain8/1 -> Switch3/3
  Clock1/1 -> Switch3/2

== system DEF_2GFL_Eugenie/DEF_DualFrictionYunjie3/Initial_filter2 ==
  original : Inport
  Clock1 : Clock
  Gain7 : Gain
  Gain8 : Gain  Gain=0
  Switch3 : Switch  Criteria=u2 > Threshold  Threshold=1.5  SaturateOnIntegerOverflow=off  InputSameDT=off
  filtered : Outport
  wires:
  Switch3/1 -> filtered/1  "dTheta"
  original/1 -> Gain8/1, Gain7/1
  Gain7/1 -> Switch3/1
  Gain8/1 -> Switch3/3
  Clock1/1 -> Switch3/2

== system DEF_2GFL_Eugenie/DEF_DualFrictionYunjie3/Initial_filter3 ==
  original : Inport
  Clock1 : Clock
  Gain7 : Gain
  Gain8 : Gain  Gain=0
  Switch3 : Switch  Criteria=u2 > Threshold  Threshold=1.5  SaturateOnIntegerOverflow=off  InputSameDT=off
  filtered : Outport
  wires:
  Switch3/1 -> filtered/1  "dTheta"
  original/1 -> Gain8/1, Gain7/1
  Gain7/1 -> Switch3/1
  Gain8/1 -> Switch3/3
  Clock1/1 -> Switch3/2

== system DEF_2GFL_Eugenie/DEF_Friction1/Initial_filter ==
  original : Inport
  Clock1 : Clock
  Gain7 : Gain
  Gain8 : Gain  Gain=0
  Switch3 : Switch  Criteria=u2 > Threshold  Threshold=1.5  SaturateOnIntegerOverflow=off  InputSameDT=off
  filtered : Outport
  wires:
  Clock1/1 -> Switch3/2
  Gain8/1 -> Switch3/3
  Gain7/1 -> Switch3/1
  original/1 -> Gain7/1, Gain8/1
  Switch3/1 -> filtered/1  "dTheta"

== system DEF_2GFL_Eugenie/DEF_Friction1/Initial_filter1 ==
  original : Inport
  Clock1 : Clock
  Gain7 : Gain
  Gain8 : Gain  Gain=0
  Switch3 : Switch  Criteria=u2 > Threshold  Threshold=1.5  SaturateOnIntegerOverflow=off  InputSameDT=off
  filtered : Outport
  wires:
  Clock1/1 -> Switch3/2
  Gain8/1 -> Switch3/3
  Gain7/1 -> Switch3/1
  original/1 -> Gain7/1, Gain8/1
  Switch3/1 -> filtered/1  "dTheta"

== system DEF_2GFL_Eugenie/DEF_Friction1/Initial_filter2 ==
  original : Inport
  Clock1 : Clock
  Gain7 : Gain
  Gain8 : Gain  Gain=0
  Switch3 : Switch  Criteria=u2 > Threshold  Threshold=1.5  SaturateOnIntegerOverflow=off  InputSameDT=off
  filtered : Outport
  wires:
  Clock1/1 -> Switch3/2
  Gain8/1 -> Switch3/3
  Gain7/1 -> Switch3/1
  original/1 -> Gain7/1, Gain8/1
  Switch3/1 -> filtered/1  "dTheta"

== system DEF_2GFL_Eugenie/DEF_Friction1/Initial_filter3 ==
  original : Inport
  Clock1 : Clock
  Gain7 : Gain
  Gain8 : Gain  Gain=0
  Switch3 : Switch  Criteria=u2 > Threshold  Threshold=1.5  SaturateOnIntegerOverflow=off  InputSameDT=off
  filtered : Outport
  wires:
  Clock1/1 -> Switch3/2
  Gain8/1 -> Switch3/3
  Gain7/1 -> Switch3/1
  original/1 -> Gain7/1, Gain8/1
  Switch3/1 -> filtered/1  "dTheta"

== system DEF_2GFL_Eugenie/DEF_Friction2/Initial_filter ==
  original : Inport
  Clock1 : Clock
  Gain7 : Gain
  Gain8 : Gain  Gain=0
  Switch3 : Switch  Criteria=u2 > Threshold  Threshold=1.5  SaturateOnIntegerOverflow=off  InputSameDT=off
  filtered : Outport
  wires:
  Clock1/1 -> Switch3/2
  Gain8/1 -> Switch3/3
  Gain7/1 -> Switch3/1
  original/1 -> Gain7/1, Gain8/1
  Switch3/1 -> filtered/1  "dTheta"

== system DEF_2GFL_Eugenie/DEF_Friction2/Initial_filter1 ==
  original : Inport
  Clock1 : Clock
  Gain7 : Gain
  Gain8 : Gain  Gain=0
  Switch3 : Switch  Criteria=u2 > Threshold  Threshold=1.5  SaturateOnIntegerOverflow=off  InputSameDT=off
  filtered : Outport
  wires:
  Clock1/1 -> Switch3/2
  Gain8/1 -> Switch3/3
  Gain7/1 -> Switch3/1
  original/1 -> Gain7/1, Gain8/1
  Switch3/1 -> filtered/1  "dTheta"

== system DEF_2GFL_Eugenie/DEF_Friction2/Initial_filter2 ==
  original : Inport
  Clock1 : Clock
  Gain7 : Gain
  Gain8 : Gain  Gain=0
  Switch3 : Switch  Criteria=u2 > Threshold  Threshold=1.5  SaturateOnIntegerOverflow=off  InputSameDT=off
  filtered : Outport
  wires:
  Clock1/1 -> Switch3/2
  Gain8/1 -> Switch3/3
  Gain7/1 -> Switch3/1
  original/1 -> Gain7/1, Gain8/1
  Switch3/1 -> filtered/1  "dTheta"

== system DEF_2GFL_Eugenie/DEF_Friction2/Initial_filter3 ==
  original : Inport
  Clock1 : Clock
  Gain7 : Gain
  Gain8 : Gain  Gain=0
  Switch3 : Switch  Criteria=u2 > Threshold  Threshold=1.5  SaturateOnIntegerOverflow=off  InputSameDT=off
  filtered : Outport
  wires:
  Clock1/1 -> Switch3/2
  Gain8/1 -> Switch3/3
  Gain7/1 -> Switch3/1
  original/1 -> Gain7/1, Gain8/1
  Switch3/1 -> filtered/1  "dTheta"

== system DEF_2GFL_Eugenie/VSI-PLL2/FO ==
  Vd : Inport
  Divide : Product  Inputs=**
  Divide1 : Product  Inputs=**
  Gain4 : Gain  Gain=0
  Sine Wave : Sin  Frequency=2*pi*3  SampleTime=0
  Step : Step  Time=2  SampleTime=0
  Out1 : Outport
  wires:
  Vd/1 -> Gain4/1
  Sine Wave/1 -> Divide/2
  Step/1 -> Divide1/2
  Divide/1 -> Divide1/1
  Divide1/1 -> Out1/1
  Gain4/1 -> Divide/1

== system DEF_2GFL_Eugenie/VSI-PLL2/Forced oscillation ==
  Vd : Inport
  Divide : Product  Inputs=**
  Divide1 : Product  Inputs=**
  Gain4 : Gain  Gain=0.02
  Sine Wave : Sin  Frequency=2*pi*3  SampleTime=0
  Step : Step  Time=2  SampleTime=0
  Out1 : Outport
  wires:
  Gain4/1 -> Divide/1
  Divide1/1 -> Out1/1
  Divide/1 -> Divide1/1
  Step/1 -> Divide1/2
  Sine Wave/1 -> Divide/2
  Vd/1 -> Gain4/1

== system DEF_2GFL_Eugenie/VSI-PLL2/Forced oscillation1 ==
  Vq : Inport
  Constant : Constant
  Divide : Product  Inputs=**
  Divide1 : Product  Inputs=**
  Gain4 : Gain  Gain=0
  Sine Wave : Sin  Frequency=2*pi*3  Phase=pi  SampleTime=0
  Step : Step  Time=2  SampleTime=0
  Out1 : Outport
  wires:
  Constant/1 -> Gain4/1
  Sine Wave/1 -> Divide/2
  Step/1 -> Divide1/2
  Divide/1 -> Divide1/1
  Divide1/1 -> Out1/1
  Gain4/1 -> Divide/1
